simulink subsystem "missile_position_subsystem"  (R2021b)
settings: Solver=VariableStepAuto  StartTime=0.0  StopTime=10.0  RelTol=1e-3
values from neighbouring files (symbols this model uses):
  X_M0 = 2000    [PN_Guidance_matlab.m]
  Z_M0 = 0    [PN_Guidance_matlab.m]
settings Model: Creator=rocke  LastModifiedBy=rocke

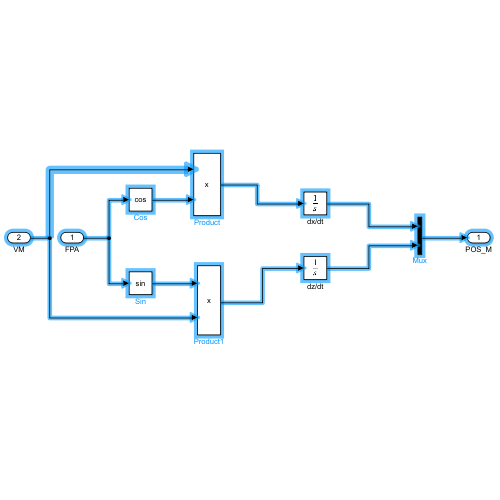
[thumbnail: Simulink's stored preview of the top-level diagram]
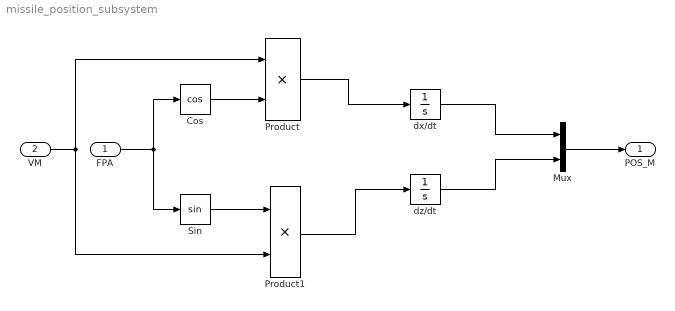
== system missile_position_subsystem ==
  FPA : Inport
  VM : Inport  Port=2
  Cos : Trigonometry  Operator=cos
  Mux : Mux  Inputs=2
  Product : Product
  Product1 : Product
  Sin : Trigonometry
  dx/dt : Integrator  InitialCondition=X_M0
  dz/dt : Integrator  InitialCondition=Z_M0
  POS_M : Outport
  wires:
  Product1/1 -> dz/dt/1
  Product/1 -> dx/dt/1
  dz/dt/1 -> Mux/2
  Cos/1 -> Product/2
  dx/dt/1 -> Mux/1
  Sin/1 -> Product1/1
  FPA/1 -> Sin/1, Cos/1
  Mux/1 -> POS_M/1
  VM/1 -> Product/1, Product1/2
